simulink library "DEM_lib"  (Simulink 7.4)
settings: Solver=FixedStepDiscrete  StartTime=0.0  StopTime=Inf  FixedStep=0.001  RelTol=1e-3
undefined symbols (not defined in the file or in its folder): BCU_Drive_St, BCU_FastCharge_St, BCU_SlowCharge_St, COR_Fault_Bus, CTC_DefaultOffline_CtrCmd, CTC_DriveEmgyDcnct_CtrCmd, CTC_DriveOffline_CtrCmd, CTC_DriveOnline_CtrCmd, EHP_Fault_Bus, FCM_Fault_Bus, SCM_Fault_Bus
libraries: Defined_Functionality x82, simulink x2
(part 1 of 4)
Description:
  | $Author:Yan LiJuan$
  | $Date:2015/03/26$
  | $Revision:1.0$
settings Model: Creator=yanlijuan2  LastModifiedBy=sunsijun

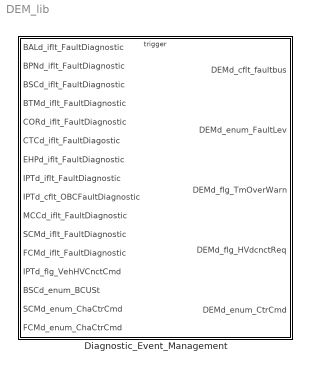
== system DEM_lib ==
  Diagnostic_Event_Management : Subsystem  TreatAsAtomicUnit=on

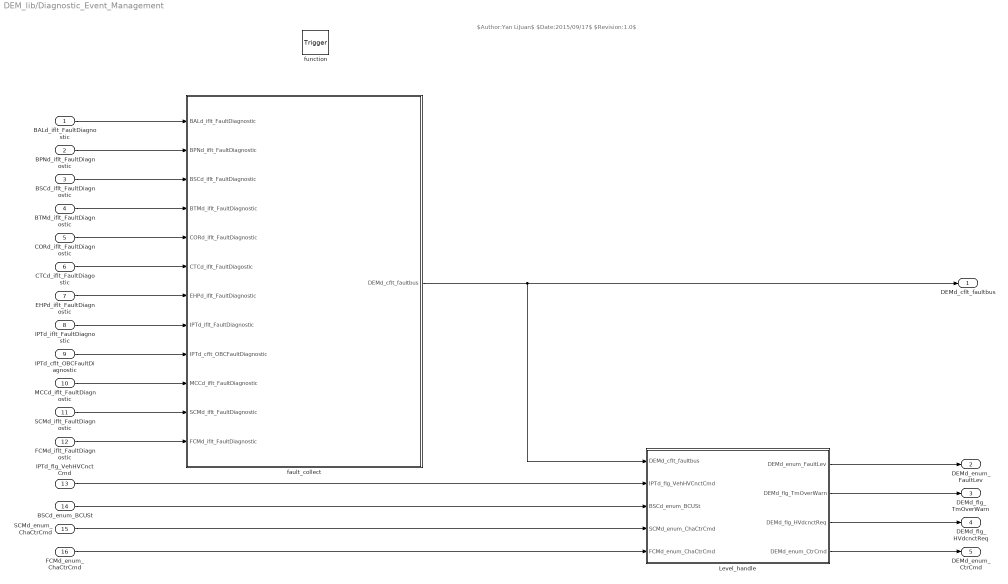
== system DEM_lib/Diagnostic_Event_Management ==
  note: $Author:Yan LiJuan$
      | $Date:2015/09/17$
      | $Revision:1.0$
  BALd_iflt_FaultDiagnostic : Inport
  BPNd_iflt_FaultDiagnostic : Inport  Port=2
  BSCd_iflt_FaultDiagnostic : Inport  Port=3
  BTMd_iflt_FaultDiagnostic : Inport  Port=4
  CORd_iflt_FaultDiagnostic : Inport  Port=5
  CTCd_iflt_FaultDiagostic : Inport  Port=6
  EHPd_iflt_FaultDiagnostic : Inport  Port=7
  IPTd_iflt_FaultDiagnostic : Inport  Port=8
  IPTd_cflt_OBCFaultDiagnostic : Inport  Port=9
  MCCd_iflt_FaultDiagnostic : Inport  Port=10
  SCMd_iflt_FaultDiagnostic : Inport  Port=11
  FCMd_iflt_FaultDiagnostic : Inport  Port=12
  IPTd_flg_VehHVCnctCmd : Inport  Port=13  DataType=boolean  OutDataTypeStr=boolean
  BSCd_enum_BCUSt : Inport  Port=14  DataType=uint8  OutDataTypeStr=uint8
  SCMd_enum_ChaCtrCmd : Inport  Port=15  DataType=uint8  OutDataTypeStr=uint8
  FCMd_enum_ChaCtrCmd : Inport  Port=16  DataType=uint8  OutDataTypeStr=uint8
  function : TriggerPort  TriggerType=function-call
  Level_handle : Subsystem  Description=|
      | $Author:Yan LiJuan$
      | $Date:2015/06/23$  
      | $Revision:1.0$
  fault_collect : Subsystem  Description=|
      | $Author:Yan LiJuan$
      | $Date:2015/06/23$  
      | $Revision:1.0$
  DEMd_cflt_faultbus : Outport  OutDataType=fixdt(1, 16)  OutScaling=2^0
  DEMd_enum_FaultLev : Outport  Port=2
  DEMd_flg_TmOverWarn : Outport  Port=3
  DEMd_flg_HVdcnctReq : Outport  Port=4
  DEMd_enum_CtrCmd : Outport  Port=5
  wires:
  IPTd_cflt_OBCFaultDiagnostic/1 -> fault_collect/9(IPTd_cflt_OBCFaultDiagnostic)
  BALd_iflt_FaultDiagnostic/1 -> fault_collect/1(BALd_iflt_FaultDiagnostic)
  BPNd_iflt_FaultDiagnostic/1 -> fault_collect/2(BPNd_iflt_FaultDiagnostic)
  BSCd_iflt_FaultDiagnostic/1 -> fault_collect/3(BSCd_iflt_FaultDiagnostic)
  BTMd_iflt_FaultDiagnostic/1 -> fault_collect/4(BTMd_iflt_FaultDiagnostic)
  CORd_iflt_FaultDiagnostic/1 -> fault_collect/5(CORd_iflt_FaultDiagnostic)
  CTCd_iflt_FaultDiagostic/1 -> fault_collect/6(CTCd_iflt_FaultDiagostic)
  fault_collect/1(DEMd_cflt_faultbus) -> DEMd_cflt_faultbus/1, Level_handle/1(DEMd_cflt_faultbus)
  EHPd_iflt_FaultDiagnostic/1 -> fault_collect/7(EHPd_iflt_FaultDiagnostic)
  IPTd_iflt_FaultDiagnostic/1 -> fault_collect/8(IPTd_iflt_FaultDiagnostic)
  MCCd_iflt_FaultDiagnostic/1 -> fault_collect/10(MCCd_iflt_FaultDiagnostic)
  SCMd_iflt_FaultDiagnostic/1 -> fault_collect/11(SCMd_iflt_FaultDiagnostic)
  FCMd_iflt_FaultDiagnostic/1 -> fault_collect/12(FCMd_iflt_FaultDiagnostic)
  Level_handle/1(DEMd_enum_FaultLev) -> DEMd_enum_FaultLev/1
  Level_handle/2(DEMd_flg_TmOverWarn) -> DEMd_flg_TmOverWarn/1
  IPTd_flg_VehHVCnctCmd/1 -> Level_handle/2(IPTd_flg_VehHVCnctCmd)
  Level_handle/3(DEMd_flg_HVdcnctReq) -> DEMd_flg_HVdcnctReq/1
  BSCd_enum_BCUSt/1 -> Level_handle/3(BSCd_enum_BCUSt)
  Level_handle/4(DEMd_enum_CtrCmd) -> DEMd_enum_CtrCmd/1
  SCMd_enum_ChaCtrCmd/1 -> Level_handle/4(SCMd_enum_ChaCtrCmd)
  FCMd_enum_ChaCtrCmd/1 -> Level_handle/5(FCMd_enum_ChaCtrCmd)

== system DEM_lib/Diagnostic_Event_Management/Level_handle ==
  DEMd_cflt_faultbus : Inport
  IPTd_flg_VehHVCnctCmd : Inport  Port=2  DataType=boolean  OutDataTypeStr=boolean
  BSCd_enum_BCUSt : Inport  Port=3  DataType=uint8  OutDataTypeStr=uint8
  SCMd_enum_ChaCtrCmd : Inport  Port=4  DataType=uint8  OutDataTypeStr=uint8
  FCMd_enum_ChaCtrCmd : Inport  Port=5  DataType=uint8  OutDataTypeStr=uint8
  CtrCmdSelect : Subsystem  Description=|
      | $Author:Yan LiJuan$
      | $Date:2015/03/26$  
      | $Revision:1.0$
  DRIVE : Subsystem  Description=|
      | $Author:Yan LiJuan$
      | $Date:2015/03/26$  
      | $Revision:1.0$
  DEMd_enum_FaultLev : Outport
  DEMd_flg_TmOverWarn : Outport  Port=2
  DEMd_flg_HVdcnctReq : Outport  Port=3
  DEMd_enum_CtrCmd : Outport  Port=4
  wires:
  DRIVE/3(DEMd_flg_HVdcnctReq) -> DEMd_flg_HVdcnctReq/1
  DRIVE/4(DEMd_enum_DrvCtrCmdRaw) -> CtrCmdSelect/1(DEMd_enum_DrvCtrCmd)
  DRIVE/2(DEMd_flg_TmOverWarn) -> DEMd_flg_TmOverWarn/1
  FCMd_enum_ChaCtrCmd/1 -> CtrCmdSelect/4(FCHMd_enum_ChaCtrCmd)
  SCMd_enum_ChaCtrCmd/1 -> CtrCmdSelect/3(SCMd_enum_ChaCtrCmd)
  CtrCmdSelect/1(DEMd_enum_CtrCmd) -> DEMd_enum_CtrCmd/1
  DRIVE/1(DEMd_enum_FaultLev) -> DEMd_enum_FaultLev/1
  BSCd_enum_BCUSt/1 -> DRIVE/3(BSCd_enum_BCUSt), CtrCmdSelect/2(BSCd_enum_BCUSt)
  IPTd_flg_VehHVCnctCmd/1 -> DRIVE/2(IPTd_flg_VehHVCnctCmd)
  DEMd_cflt_faultbus/1 -> DRIVE/1(DEMd_cflt_fault)

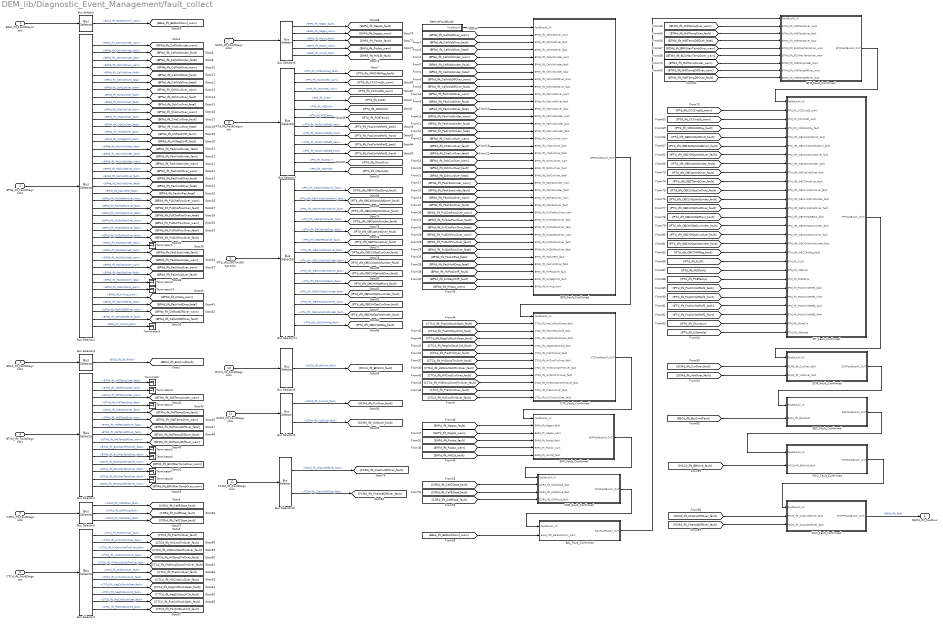
== system DEM_lib/Diagnostic_Event_Management/fault_collect ==
  BALd_iflt_FaultDiagnostic : Inport
  BPNd_iflt_FaultDiagnostic : Inport  Port=2
  BSCd_iflt_FaultDiagnostic : Inport  Port=3
  BTMd_iflt_FaultDiagnostic : Inport  Port=4
  CORd_iflt_FaultDiagnostic : Inport  Port=5
  CTCd_iflt_FaultDiagostic : Inport  Port=6
  EHPd_iflt_FaultDiagnostic : Inport  Port=7
  IPTd_iflt_FaultDiagnostic : Inport  Port=8
  IPTd_cflt_OBCFaultDiagnostic : Inport  Port=9
  MCCd_iflt_FaultDiagnostic : Inport  Port=10
  SCMd_iflt_FaultDiagnostic : Inport  Port=11
  FCMd_iflt_FaultDiagnostic : Inport  Port=12
  BAL_Fault_Confirmed : Subsystem  Description=|
      | $Author:Yan LiJuan$
      | $Date:2015/03/26$  
      | $Revision:1.0$
  BPN_Fault_Confirmed : Subsystem  Description=|
      | $Author:Yan LiJuan$
      | $Date:2015/03/26$  
      | $Revision:1.0$
  BSC_Fault_Confirmed : Subsystem  Description=|
      | $Author:Yan LiJuan$
      | $Date:2015/03/26$  
      | $Revision:1.0$
  BTM_Fault_Confirmed : Subsystem  Description=|
      | $Author:Yan LiJuan$
      | $Date:2015/03/26$  
      | $Revision:1.0$
  Bus Selector : BusSelector  OutputSignals=BALd_iflt_BalSwthAnml_warn
  Bus Selector1 : BusSelector  OutputSignals=CTCd_iflt_PrecTmOver_fault,CTCd_iflt_HVCnctTmOver_fault,CTCd_iflt_HVDcncWaitTmOver_fault,CTCd_iflt_HVDcnctTmOver_fault,CTCd_iflt_HVEmcyDcnctTmOver_fault,CTCd_iflt_PrecCurOver_fault,CTCd_iflt_HVCnctCurOver_fault,CTCd_iflt_NegCtrStuckOpen_fault,CTCd_iflt_NegCtrStuckCld_fault,CTCd_iflt_PosCtrStuckOpen_fault,CTCd_iflt_PosCtrStuckCld_fault
  Bus Selector10 : BusSelector  OutputSignals=FCMd_iflt_ChaCurDifOver_fault,FCMd_iflt_ChaVoltDifOver_fault
  Bus Selector11 : BusSelector  OutputSignals=IPTd_cflt_OBCHVOptDcnct_fault,IPTd_cflt_OBCAVOptVoltAbnml_fault,IPTd_cflt_OBCHVOptVoltOver_fault,IPTd_cflt_OBCIptVoltUnder_fault,IPTd_cflt_OBCIptVoltOver_fault,IPTd_cflt_OBCTempOver_fault,IPTd_cflt_OBCLVOptCurOver_fault,IPTd_cflt_OBCLVOptVoltUnder_fault,IPTd_cflt_OBCLVOptVoltOver_fault,IPTd_cflt_OBCHVOptRevs_fault,IPTd_cflt_OBCHVOptCurUnder_fault,IPTd_cflt_OBCHVOptCurOver_fault,IPTd_cflt_OBCHVOptVoltUnder_fault,IPTd_cflt_OBCCANMsg_fault
  Bus Selector2 : BusSelector  OutputSignals=BPNd_iflt_CellVoltDiag.BPNd_iflt_CellVoltUnder_warn,BPNd_iflt_CellVoltDiag.BPNd_iflt_CellVoltUnder_fault,BPNd_iflt_CellVoltDiag.BPNd_iflt_CellVoltUnder_fatal,BPNd_iflt_CellVoltDiag.BPNd_iflt_CellVoltOver_warn,BPNd_iflt_CellVoltDiag.BPNd_iflt_CellVoltOver_fault,BPNd_iflt_CellVoltDiag.BPNd_iflt_CellVoltOver_fatal,BPNd_iflt_ActCurDiag.BPNd_iflt_DchCurOver_warn,BPNd_iflt_ActCurDiag.BPNd_iflt_DchCurOver_fault,BPNd_iflt_ActCurDiag.BPNd_iflt_DchCurOver_fatal,BPNd_iflt_ActCurDiag.BPNd_iflt_ChaCurOver_warn,BPNd_iflt_ActCurDiag.BPNd_iflt_ChaCurOver_fault,BPNd_iflt_ActCurDiag.BPNd_iflt_ChaCurOver_fatal,BPNd_iflt_HVCtrRDiag.BPNd_iflt_HVPosCtrlR_fault,BPNd_iflt_HVCtrRDiag.BPNd_iflt_HVNegCtrlR_fault,BPNd_iflt_HighVoltDiag.BPNd_iflt_PackVoltUnder_fatal,BPNd_iflt_HighVoltDiag.BPNd_iflt_PackVoltUnder_fault,BPNd_iflt_HighVoltDiag.BPNd_iflt_PackVoltUnder_warn,BPNd_iflt_HighVoltDiag.BPNd_iflt_PackVoltOver_warn,BPNd_iflt_HighVoltDiag.BPNd_iflt_PackVoltOver_fault,BPNd_iflt_HighVoltDiag.BPNd_iflt_PackVoltOver_fatal,BPNd_iflt_PackInResDiag.BPNd_iflt_PackInRes_fatal,BPNd_iflt_ActPowDiag.BPNd_iflt_PulChaPowOver_warn,BPNd_iflt_ActPowDiag.BPNd_iflt_PulChaPowOver_fault,BPNd_iflt_ActPowDiag.BPNd_iflt_PulChaPowOver_fatal,BPNd_iflt_ActPowDiag.BPNd_iflt_PulDchPowOver_warn,BPNd_iflt_ActPowDiag.BPNd_iflt_PulDchPowOver_fatal,BPNd_iflt_ActPowDiag.BPNd_iflt_PulDchPowOver_fault,BPNd_iflt_SOCDiag.BPNd_iflt_PackSocUnder_fatal,BPNd_iflt_SOCDiag.BPNd_iflt_PackSocUnder_fault,BPNd_iflt_SOCDiag.BPNd_iflt_PackSocUnder_warn,BPNd_iflt_SOCDiag.BPNd_iflt_PackSocOver_warn,BPNd_iflt_SOCDiag.BPNd_iflt_PackSocOver_fault,BPNd_iflt_SOCDiag.BPNd_iflt_PackSocOver_fatal,BPNd_iflt_VoltAcqDiag.BPNd_iflt_MSDVoltAcq_warn,BPNd_iflt_VoltAcqDiag.BPNd_iflt_HVAcq_warn,BPNd_ilft_PackVoltDropDiag.BPNd_ilft_PackVoltDrop_fatal,BPNd_iflt_CellVoltDifDiag.BPNd_iflt_CellVoltDifOver_warn,BPNd_iflt_CellVoltDifDiag.BPNd_iflt_CellVoltDifOver_fault,BPNd_iflt_CurAcqDiag.BPNd_iflt_CurAcq_fault
  Bus Selector3 : BusSelector  OutputSignals=BSCd_iflt_BCUFault
  Bus Selector4 : BusSelector  OutputSignals=BTMd_iflt_MdlTempUnder_fatal,BTMd_iflt_MdlTempUnder_fault,BTMd_iflt_MdlTempUnder_warn,BTMd_iflt_MdlTempOver_fatal,BTMd_iflt_MdlTempOver_fault,BTMd_iflt_MdlTempOver_warn,BTMd_iflt_MdlTempDifOver_fatal,BTMd_iflt_MdlTempDifOver_fault,BTMd_iflt_MdlTempDifOver_warn,BTMd_iflt_BCUMaxTempOver_fatal,BTMd_iflt_BCUMaxTempOver_fault,BTMd_iflt_BCUMaxTempOver_warn,BTMd_iflt_BMUMaxTempOver_fatal,BTMd_iflt_BMUMaxTempOver_fault,BTMd_iflt_BMUMaxTempOver_warn
  Bus Selector5 : BusSelector  OutputSignals=CORd_iflt_CellRDcse_fault,CORd_iflt_CellRIcse_fault,CORd_iflt_CellCDcse_fault
  Bus Selector6 : BusSelector  OutputSignals=EHPd_iflt_NegIso_fault,EHPd_iflt_NegIso_warn,EHPd_iflt_PosIso_fault,EHPd_iflt_PosIso_warn,EHPd_iflt_HVILSt_fault
  Bus Selector7 : BusSelector  OutputSignals=IPTd_iflt_VMSCANMsg_fault,IPTd_iflt_CC2CnctSt_warn,IPTd_iflt_CCCnctSt_warn,IPTd_iflt_AnalogDiagnostic.IPTd_iflt_KL30,IPTd_iflt_AnalogDiagnostic.IPTd_iflt_MSDVolt,IPTd_iflt_AnalogDiagnostic.IPTd_iflt_PCBTemp,IPTd_iflt_AnalogDiagnostic.IPTd_iflt_PosCtrVoltRef1_back,IPTd_iflt_AnalogDiagnostic.IPTd_iflt_PosCtrVoltRef1_front,IPTd_iflt_AnalogDiagnostic.IPTd_iflt_PosCtrVoltRef2_back,IPTd_iflt_AnalogDiagnostic.IPTd_iflt_PosCtrVoltRef2_front,IPTd_iflt_AnalogDiagnostic.IPTd_iflt_ShuntCur,IPTd_iflt_AnalogDiagnostic.IPTd_iflt_USample
  Bus Selector8 : BusSelector  OutputSignals=MCCd_iflt_BMUInit_fault
  Bus Selector9 : BusSelector  OutputSignals=SCMd_iflt_CurOver_fault,SCMd_iflt_VoltOver_fault
  COR_Fault_Confirmed : Subsystem  Description=|
      | $Author:Yan LiJuan$
      | $Date:2015/03/26$  
      | $Revision:1.0$
  CTC_Fault_Confirmed : Subsystem  Description=|
      | $Author:Yan LiJuan$
      | $Date:2015/03/26$  
      | $Revision:1.0$
  DefaultFaultBusAll : Subsystem  Description=|
      | $Author:Yan LiJuan$
      | $Date:2015/03/26$  
      | $Revision:1.0$
  EHP_Fault_Confirmed : Subsystem  Description=|
      | $Author:Yan LiJuan$
      | $Date:2015/03/26$  
      | $Revision:1.0$
  FCM_Fault_Confirmed : Subsystem  Description=|
      | $Author:Yan LiJuan$
      | $Date:2015/03/26$  
      | $Revision:1.0$
  IPT_Fault_Confirmed : Subsystem  Description=|
      | $Author:Yan LiJuan$
      | $Date:2015/03/26$  
      | $Revision:1.0$
  MCC_Fault_Confirmed : Subsystem  Description=|
      | $Author:Yan LiJuan$
      | $Date:2015/03/26$  
      | $Revision:1.0$
  SCM_Fault_Confirmed : Subsystem  Description=|
      | $Author:Yan LiJuan$
      | $Date:2015/03/26$  
      | $Revision:1.0$
  Terminator{,1..10} (11 alike) : Terminator
  DEMd_cflt_faultbus : Outport  OutDataType=fixdt(1, 16)  OutScaling=2^0
  wires:
  Bus Selector2/39 -> Terminator9/1  "<BPNd_iflt_CurAcq_fault>"
  Bus Selector2/35 -> [BPNd_iflt_HVAcq_warn]  "<BPNd_iflt_HVAcq_warn>"
  [IPTd_cflt_OBCHVOptDcnct_fault] -> IPT_Fault_Confirmed/5(IPTd_cflt_OBCHVOptDcnct_fault)
  [IPTd_cflt_OBCAVOptVoltAbnml_fault] -> IPT_Fault_Confirmed/6(IPTd_cflt_OBCAVOptVoltAbnml_fault)
  Bus Selector11/14 -> [IPTd_cflt_OBCCANMsg_fault]  "<IPTd_cflt_OBCCANMsg_fault>"
  Bus Selector11/13 -> [IPTd_cflt_OBCHVOptVoltUnder_fault]  "<IPTd_cflt_OBCHVOptVoltUnder_fault>"
  Bus Selector11/12 -> [IPTd_cflt_OBCHVOptCurOver_fault]  "<IPTd_cflt_OBCHVOptCurOver_fault>"
  Bus Selector11/11 -> [IPTd_cflt_OBCHVOptCurUnder_fault]  "<IPTd_cflt_OBCHVOptCurUnder_fault>"
  Bus Selector11/10 -> [IPTd_cflt_OBCHVOptRevs_fault]  "<IPTd_cflt_OBCHVOptRevs_fault>"
  Bus Selector11/9 -> [IPTd_cflt_OBCLVOptVoltOver_fault]  "<IPTd_cflt_OBCLVOptVoltOver_fault>"
  Bus Selector11/8 -> [IPTd_cflt_OBCLVOptVoltUnder_fault]  "<IPTd_cflt_OBCLVOptVoltUnder_fault>"
  Bus Selector11/7 -> [IPTd_cflt_OBCLVOptCurOver_fault]  "<IPTd_cflt_OBCLVOptCurOver_fault>"
  Bus Selector11/6 -> [IPTd_cflt_OBCTempOver_fault]  "<IPTd_cflt_OBCTempOver_fault>"
  Bus Selector11/5 -> [IPTd_cflt_OBCIptVoltOver_fault]  "<IPTd_cflt_OBCIptVoltOver_fault>"
  Bus Selector11/4 -> [IPTd_cflt_OBCIptVoltUnder_fault]  "<IPTd_cflt_OBCIptVoltUnder_fault>"
  Bus Selector11/3 -> [IPTd_cflt_OBCHVOptVoltOver_fault]  "<IPTd_cflt_OBCHVOptVoltOver_fault>"
  Bus Selector11/2 -> [IPTd_cflt_OBCAVOptVoltAbnml_fault]  "<IPTd_cflt_OBCAVOptVoltAbnml_fault>"
  Bus Selector11/1 -> [IPTd_cflt_OBCHVOptDcnct_fault]  "<IPTd_cflt_OBCHVOptDcnct_fault>"
  Bus Selector7/12 -> [IPTd_iflt_USample]  "<IPTd_iflt_USample>"
  Bus Selector7/11 -> [IPTd_iflt_ShuntCur]  "<IPTd_iflt_ShuntCur>"
  Bus Selector7/10 -> [IPTd_iflt_PosCtrVoltRef2_front]  "<IPTd_iflt_PosCtrVoltRef2_front>"
  Bus Selector7/9 -> [IPTd_iflt_PosCtrVoltRef2_back]  "<IPTd_iflt_PosCtrVoltRef2_back>"
  Bus Selector7/8 -> [IPTd_iflt_PosCtrVoltRef1_front]  "<IPTd_iflt_PosCtrVoltRef1_front>"
  Bus Selector7/7 -> [IPTd_iflt_PosCtrVoltRef1_back]  "<IPTd_iflt_PosCtrVoltRef1_back>"
  Bus Selector7/6 -> [IPTd_iflt_PCBTemp]  "<IPTd_iflt_PCBTemp>"
  Bus Selector7/5 -> [IPTd_iflt_MSDVolt]  "<IPTd_iflt_MSDVolt>"
  Bus Selector7/4 -> [IPTd_iflt_KL30]  "<IPTd_iflt_KL30>"
  Bus Selector7/3 -> [IPTd_iflt_CCCnctSt_warn]  "<IPTd_iflt_CCCnctSt_warn>"
  Bus Selector7/2 -> [IPTd_iflt_CC2CnctSt_warn]  "<IPTd_iflt_CC2CnctSt_warn>"
  Bus Selector7/1 -> [IPTd_iflt_VMSCANMsg_fault]  "<IPTd_iflt_VMSCANMsg_fault>"
  IPTd_cflt_OBCFaultDiagnostic/1 -> Bus Selector11/1
  FCM_Fault_Confirmed/1(FCMIPTFaultBusAll_OUT) -> DEMd_cflt_faultbus/1  "DEMd_cflt_fault"
  [FCMd_iflt_ChaVoltDifOver_fault] -> FCM_Fault_Confirmed/3(FCMd_iflt_ChaVoltDifOver_fault)
  [FCMd_iflt_ChaCurDifOver_fault] -> FCM_Fault_Confirmed/2(FCMd_iflt_ChaCurDifOver_fault)
  Bus Selector10/2 -> [FCMd_iflt_ChaVoltDifOver_fault]  "<FCMd_iflt_ChaVoltDifOver_fault>"
  Bus Selector10/1 -> [FCMd_iflt_ChaCurDifOver_fault]  "<FCMd_iflt_ChaCurDifOver_fault>"
  FCMd_iflt_FaultDiagnostic/1 -> Bus Selector10/1
  [BSCd_iflt_BcuCmdFault] -> BSC_Fault_Confirmed/2(BSCd_iflt_BCUFault)
  BSC_Fault_Confirmed/1(BSCFaultBusAll_OUT) -> MCC_Fault_Confirmed/1(FaultBusAll_IN)
  SCM_Fault_Confirmed/1(SCMFaultBusAll_OUT) -> BSC_Fault_Confirmed/1(FaultBusAll_IN)
  [SCMd_iflt_VoltOver_fault] -> SCM_Fault_Confirmed/3(SCMd_iflt_VoltOver_fault)
  [SCMd_iflt_CurOver_fault] -> SCM_Fault_Confirmed/2(SCMd_iflt_CurOver_fault)
  Bus Selector9/2 -> [SCMd_iflt_VoltOver_fault]  "<SCMd_iflt_VoltOver_fault>"
  SCMd_iflt_FaultDiagnostic/1 -> Bus Selector9/1
  Bus Selector9/1 -> [SCMd_iflt_CurOver_fault]  "<SCMd_iflt_CurOver_fault>"
  [IPTd_cflt_OBCCANMsg_fault] -> IPT_Fault_Confirmed/18(IPTd_cflt_OBCCANMsg_fault)
  [IPTd_cflt_OBCHVOptVoltUnder_fault] -> IPT_Fault_Confirmed/17(IPTd_cflt_OBCHVOptVoltUnder_fault)
  [IPTd_cflt_OBCHVOptCurOver_fault] -> IPT_Fault_Confirmed/16(IPTd_cflt_OBCHVOptCurOver_fault)
  [IPTd_cflt_OBCHVOptCurUnder_fault] -> IPT_Fault_Confirmed/15(IPTd_cflt_OBCHVOptCurUnder_fault)
  [IPTd_cflt_OBCHVOptRevs_fault] -> IPT_Fault_Confirmed/14(IPTd_cflt_OBCHVOptRevs_fault)
  [IPTd_cflt_OBCLVOptVoltOver_fault] -> IPT_Fault_Confirmed/13(IPTd_cflt_OBCLVOptVoltOver_fault)
  [IPTd_cflt_OBCLVOptVoltUnder_fault] -> IPT_Fault_Confirmed/12(IPTd_cflt_OBCLVOptVoltUnder_fault)
  [IPTd_cflt_OBCLVOptCurOver_fault] -> IPT_Fault_Confirmed/11(IPTd_cflt_OBCLVOptCurOver_fault)
  [IPTd_cflt_OBCTempOver_fault] -> IPT_Fault_Confirmed/10(IPTd_cflt_OBCTempOver_fault)
  [IPTd_cflt_OBCIptVoltOver_fault] -> IPT_Fault_Confirmed/9(IPTd_cflt_OBCIptVoltOver_fault)
  [IPTd_cflt_OBCIptVoltUnder_fault] -> IPT_Fault_Confirmed/8(IPTd_cflt_OBCIptVoltUnder_fault)
  [IPTd_cflt_OBCHVOptVoltOver_fault] -> IPT_Fault_Confirmed/7(IPTd_cflt_OBCHVOptVoltOver_fault)
  [CTCd_iflt_HVCnctCurOver_fault] -> CTC_Fault_Confirmed/9(CTCd_iflt_HVDcnctTmOver_fault)
  [CTCd_iflt_HVCnctTmOver_fault] -> CTC_Fault_Confirmed/12(CTCd_iflt_HVCnctCurOver_fault)
  [CTCd_iflt_PrecCurOver_fault] -> CTC_Fault_Confirmed/11(CTCd_iflt_PrecCurOver_fault)
  [CTCd_iflt_HVEmcyDcnctTmOver_fault] -> CTC_Fault_Confirmed/10(CTCd_iflt_HVEmcyDcnctTmOver_fault)
  [CTCd_iflt_HVDcncWaitTmOver_fault] -> CTC_Fault_Confirmed/8(CTCd_iflt_HVDcncWaitTmOver_fault)
  [CTCd_iflt_HVDcnctTmOver_fault] -> CTC_Fault_Confirmed/7(CTCd_iflt_HVCnctTmOver_fault)
  [CTCd_iflt_PrecTmOver_fault] -> CTC_Fault_Confirmed/6(CTCd_iflt_PrecTmOver_fault)
  [CTCd_iflt_NegCtrStuckCld_fault] -> CTC_Fault_Confirmed/5(CTCd_iflt_NegCtrStuckCld_fault)
  [CTCd_iflt_NegCtrStuckOpen_fault] -> CTC_Fault_Confirmed/4(CTCd_iflt_NegCtrStuckOpen_fault)
  [CTCd_iflt_PosCtrStuckCld_fault] -> CTC_Fault_Confirmed/3(CTCd_iflt_PosCtrStuckCld_fault)
  [CTCd_iflt_PosCtrStuckOpen_fault] -> CTC_Fault_Confirmed/2(CTCd_iflt_PosCtrStuckOpen_fault)
  [BTMd_iflt_MdlTempUnder_warn] -> BTM_Fault_Confirmed/7(BTMd_iflt_MdlTempUnder_warn)
  [BTMd_iflt_BMUMaxTempOver_warn] -> BTM_Fault_Confirmed/5(BTMd_iflt_BMUMaxTempOver_warn)
  [BTMd_iflt_BCUMaxTempOver_warn] -> BTM_Fault_Confirmed/6(BTMd_iflt_BCUMaxTempOver_warn)
  [BTMd_iflt_MdlTempDifOver_fatal] -> BTM_Fault_Confirmed/4(BTMd_iflt_MdlTempOver_fatal)
  [BTMd_iflt_MdlTempOver_fault] -> BTM_Fault_Confirmed/3(BTMd_iflt_MdlTempOver_fault)
  [BTMd_iflt_MdlTempOver_warn] -> BTM_Fault_Confirmed/2(BTMd_iflt_MdlTempOver_warn)
  [EHPd_iflt_HVILSt_fault] -> EHP_Fault_Confirmed/6(EHPd_iflt_HVILSt_fault)
  IPT_Fault_Confirmed/1(IPTFaultBusAll_OUT) -> SCM_Fault_Confirmed/1(FaultBusAll_IN)
  BTM_Fault_Confirmed/1(BTMFaultBusAll_OUT) -> IPT_Fault_Confirmed/1(FaultBusAll_IN)
  BAL_Fault_Confirmed/1(BALFaultBusAll_OUT) -> BTM_Fault_Confirmed/1(FaultBusAll_IN)
  COR_Fault_Confirmed/1(CORFaultBusAll_OUT) -> BAL_Fault_Confirmed/1(FaultBusAll_IN)
  EHP_Fault_Confirmed/1(EHPFaultBusAll_OUT) -> COR_Fault_Confirmed/1(FaultBusAll_IN)
  [BALd_iflt_BalSwthAnml_warn] -> BAL_Fault_Confirmed/2(BALd_iflit_BalSwthAnml_warn)
  BPN_Fault_Confirmed/1(BPNFaultBusAll_OUT) -> CTC_Fault_Confirmed/1(FaultBusAll_IN)
  CTC_Fault_Confirmed/1(CTCFaultBusAll_OUT) -> EHP_Fault_Confirmed/1(FaultBusAll_IN)
  DefaultFaultBusAll/1(FaultBusAll) -> BPN_Fault_Confirmed/1(FaultBusAll_IN)
  BSCd_iflt_FaultDiagnostic/1 -> Bus Selector3/1
  BTMd_iflt_FaultDiagnostic/1 -> Bus Selector4/1
  CORd_iflt_FaultDiagnostic/1 -> Bus Selector5/1
  CTCd_iflt_FaultDiagostic/1 -> Bus Selector1/1
  MCCd_iflt_FaultDiagnostic/1 -> Bus Selector8/1
  BPNd_iflt_FaultDiagnostic/1 -> Bus Selector2/1
  BALd_iflt_FaultDiagnostic/1 -> Bus Selector/1
  Bus Selector/1 -> [BALd_iflt_BalSwthAnml_warn]  "<BALd_iflt_BalSwthAnml_warn>"
  Bus Selector2/1 -> [BPNd_iflt_CellVoltUnder_warn]  "<BPNd_iflt_CellVoltUnder_warn>"
  Bus Selector2/2 -> [BPNd_iflt_CellVoltUnder_fault]  "<BPNd_iflt_CellVoltUnder_fault>"
  Bus Selector2/3 -> [BPNd_iflt_CellVoltUnder_fatal]  "<BPNd_iflt_CellVoltUnder_fatal>"
  Bus Selector2/4 -> [BPNd_iflt_CellVoltOver_warn]  "<BPNd_iflt_CellVoltOver_warn>"
  Bus Selector2/5 -> [BPNd_iflt_CellVoltOver_fault]  "<BPNd_iflt_CellVoltOver_fault>"
  Bus Selector2/6 -> [BPNd_iflt_CellVoltOver_fatal]  "<BPNd_iflt_CellVoltOver_fatal>"
  Bus Selector2/7 -> [BPNd_iflt_DchCurOver_warn]  "<BPNd_iflt_DchCurOver_warn>"
  Bus Selector2/8 -> [BPNd_iflt_DchCurOver_fault]  "<BPNd_iflt_DchCurOver_fault>"
  Bus Selector2/9 -> [BPNd_iflt_DchCurOver_fatal]  "<BPNd_iflt_DchCurOver_fatal>"
  Bus Selector2/10 -> [BPNd_iflt_ChaCurOver_warn]  "<BPNd_iflt_ChaCurOver_warn>"
  Bus Selector2/11 -> [BPNd_iflt_ChaCurOver_fault]  "<BPNd_iflt_ChaCurOver_fault>"
  Bus Selector2/12 -> [BPNd_iflt_ChaCurOver_fatal]  "<BPNd_iflt_ChaCurOver_fatal>"
  Bus Selector2/13 -> [BPNd_iflt_HVPosCtrlR_fault]  "<BPNd_iflt_HVPosCtrlR_fault>"
  Bus Selector2/14 -> [BPNd_iflt_HVNegCtrlR_fault]  "<BPNd_iflt_HVNegCtrlR_fault>"
  Bus Selector2/15 -> [BPNd_iflt_PackVoltUnder_fatal]  "<BPNd_iflt_PackVoltUnder_fatal>"
  Bus Selector2/16 -> [BPNd_iflt_PackVoltUnder_fault]  "<BPNd_iflt_PackVoltUnder_fault>"
  Bus Selector2/17 -> [BPNd_iflt_PackVoltUnder_warn]  "<BPNd_iflt_PackVoltUnder_warn>"
  Bus Selector2/18 -> [BPNd_iflt_PackVoltOver_warn]  "<BPNd_iflt_PackVoltOver_warn>"
  Bus Selector2/19 -> [BPNd_iflt_PackVoltOver_fault]  "<BPNd_iflt_PackVoltOver_fault>"
  Bus Selector2/20 -> [BPNd_iflt_PackVoltOver_fatal]  "<BPNd_iflt_PackVoltOver_fatal>"
  Bus Selector2/21 -> [BPNd_iflt_PackInRes_fatal]  "<BPNd_iflt_PackInRes_fatal>"
  Bus Selector2/22 -> [BPNd_iflt_PulChaPowOver_warn]  "<BPNd_iflt_PulChaPowOver_warn>"
  Bus Selector2/23 -> [BPNd_iflt_PulChaPowOver_fault]  "<BPNd_iflt_PulChaPowOver_fault>"
  Bus Selector2/24 -> [BPNd_iflt_PulChaPowOver_fatal]  "<BPNd_iflt_PulChaPowOver_fatal>"
  Bus Selector2/25 -> [BPNd_iflt_PulDchPowOver_warn]  "<BPNd_iflt_PulDchPowOver_warn>"
  Bus Selector2/27 -> [BPNd_iflt_PulDchPowOver_fault]  "<BPNd_iflt_PulDchPowOver_fault>"
  Bus Selector2/26 -> [BPNd_iflt_PulDchPowOver_fatal]  "<BPNd_iflt_PulDchPowOver_fatal>"
  Bus Selector2/30 -> [BPNd_iflt_PackSocUnder_warn]  "<BPNd_iflt_PackSocUnder_warn>"
  Bus Selector2/29 -> [BPNd_iflt_PackSocUnder_fault]  "<BPNd_iflt_PackSocUnder_fault>"
  Bus Selector2/28 -> Terminator1/1  "<BPNd_iflt_PackSocUnder_fatal>"
  Bus Selector2/31 -> [BPNd_iflt_PackSocOver_warn]  "<BPNd_iflt_PackSocOver_warn>"
  Bus Selector2/32 -> [BPNd_iflt_PackSocOver_fault]  "<BPNd_iflt_PackSocOver_fault>"
  Bus Selector2/33 -> Terminator2/1  "<BPNd_iflt_PackSocOver_fatal>"
  Bus Selector2/34 -> Terminator10/1  "<BPNd_iflt_MSDVoltAcq_warn>"
  Bus Selector2/36 -> [BPNd_ilft_PackVoltDrop_fatal]  "<BPNd_ilft_PackVoltDrop_fatal>"
  Bus Selector3/1 -> [BSCd_iflt_BcuCmdFault]  "<BSCd_iflt_BCUFault>"
  Bus Selector4/1 -> Terminator/1  "<BTMd_iflt_MdlTempUnder_fatal>"
  Bus Selector4/2 -> Terminator3/1  "<BTMd_iflt_MdlTempUnder_fault>"
  Bus Selector4/3 -> [BTMd_iflt_MdlTempUnder_warn]  "<BTMd_iflt_MdlTempUnder_warn>"
  Bus Selector4/4 -> Terminator4/1  "<BTMd_iflt_MdlTempOver_fatal>"
  Bus Selector4/5 -> [BTMd_iflt_MdlTempOver_fault]  "<BTMd_iflt_MdlTempOver_fault>"
  Bus Selector4/6 -> [BTMd_iflt_MdlTempOver_warn]  "<BTMd_iflt_MdlTempOver_warn>"
  Bus Selector4/7 -> [BTMd_iflt_MdlTempDifOver_fatal]  "<BTMd_iflt_MdlTempDifOver_fatal>"
  Bus Selector4/8 -> [BTMd_iflt_MdlTempDifOver_fault]  "<BTMd_iflt_MdlTempDifOver_fault>"
  Bus Selector4/9 -> [BTMd_iflt_MdlTempDifOver_warn]  "<BTMd_iflt_MdlTempDifOver_warn>"
  Bus Selector4/10 -> Terminator5/1  "<BTMd_iflt_BCUMaxTempOver_fatal>"
  Bus Selector4/11 -> Terminator6/1  "<BTMd_iflt_BCUMaxTempOver_fault>"
  Bus Selector4/12 -> [BTMd_iflt_BCUMaxTempOver_warn]  "<BTMd_iflt_BCUMaxTempOver_warn>"
  Bus Selector4/13 -> Terminator7/1  "<BTMd_iflt_BMUMaxTempOver_fatal>"
  Bus Selector4/14 -> Terminator8/1  "<BTMd_iflt_BMUMaxTempOver_fault>"
  Bus Selector4/15 -> [BTMd_iflt_BMUMaxTempOver_warn]  "<BTMd_iflt_BMUMaxTempOver_warn>"
  Bus Selector5/1 -> [CORd_iflt_CellRDcse_fault]  "<CORd_iflt_CellRDcse_fault>"
  Bus Selector5/3 -> [CORd_iflt_CellCDcse_fault]  "<CORd_iflt_CellCDcse_fault>"
  Bus Selector5/2 -> [CORd_iflt_CellRIcse_fault]  "<CORd_iflt_CellRIcse_fault>"
  Bus Selector1/1 -> [CTCd_iflt_PrecTmOver_fault]  "<CTCd_iflt_PrecTmOver_fault>"
  Bus Selector1/2 -> [CTCd_iflt_HVCnctTmOver_fault]  "<CTCd_iflt_HVCnctTmOver_fault>"
  Bus Selector1/3 -> [CTCd_iflt_HVDcncWaitTmOver_fault]  "<CTCd_iflt_HVDcncWaitTmOver_fault>"
  Bus Selector1/4 -> [CTCd_iflt_HVDcnctTmOver_fault]  "<CTCd_iflt_HVDcnctTmOver_fault>"
  Bus Selector1/5 -> [CTCd_iflt_HVEmcyDcnctTmOver_fault]  "<CTCd_iflt_HVEmcyDcnctTmOver_fault>"
  Bus Selector1/6 -> [CTCd_iflt_PrecCurOver_fault]  "<CTCd_iflt_PrecCurOver_fault>"
  Bus Selector1/7 -> [CTCd_iflt_HVCnctCurOver_fault]  "<CTCd_iflt_HVCnctCurOver_fault>"
  Bus Selector1/8 -> [CTCd_iflt_NegCtrStuckOpen_fault]  "<CTCd_iflt_NegCtrStuckOpen_fault>"
  Bus Selector1/9 -> [CTCd_iflt_NegCtrStuckCld_fault]  "<CTCd_iflt_NegCtrStuckCld_fault>"
  Bus Selector1/10 -> [CTCd_iflt_PosCtrStuckOpen_fault]  "<CTCd_iflt_PosCtrStuckOpen_fault>"
  Bus Selector1/11 -> [CTCd_iflt_PosCtrStuckCld_fault]  "<CTCd_iflt_PosCtrStuckCld_fault>"
  EHPd_iflt_FaultDiagnostic/1 -> Bus Selector6/1
  Bus Selector6/1 -> [EHPd_iflt_NegIso_fault]  "<EHPd_iflt_NegIso_fault>"
  Bus Selector6/2 -> [EHPd_iflt_NegIso_warn]  "<EHPd_iflt_NegIso_warn>"
  Bus Selector6/3 -> [EHPd_iflt_PosIso_fault]  "<EHPd_iflt_PosIso_fault>"
  Bus Selector6/4 -> [EHPd_iflt_PosIso_warn]  "<EHPd_iflt_PosIso_warn>"
  Bus Selector6/5 -> [EHPd_iflt_HVILSt_fault]  "<EHPd_iflt_HVILSt_fault>"
  IPTd_iflt_FaultDiagnostic/1 -> Bus Selector7/1
  Bus Selector8/1 -> [MCCd_iflt_BMUInit_fault]  "<MCCd_iflt_BMUInit_fault>"
  [BPNd_iflt_CellVoltOver_warn] -> BPN_Fault_Confirmed/2(BPNd_iflt_CellVoltOver_warn)
  [BPNd_iflt_CellVoltOver_fault] -> BPN_Fault_Confirmed/3(BPNd_iflt_CellVoltOver_fault)
  [BPNd_iflt_CellVoltOver_fatal] -> BPN_Fault_Confirmed/4(BPNd_iflt_CellVoltOver_fatal)
  [BPNd_iflt_CellVoltUnder_warn] -> BPN_Fault_Confirmed/5(BPNd_iflt_CellVoltUnder_warn)
  [BPNd_iflt_CellVoltUnder_fault] -> BPN_Fault_Confirmed/6(BPNd_iflt_CellVoltUnder_fault)
  [BPNd_iflt_CellVoltUnder_fatal] -> BPN_Fault_Confirmed/7(BPNd_iflt_CellVoltUnder_fatal)
  [BPNd_iflt_CellVoltDifOver_warn] -> BPN_Fault_Confirmed/8(BPNd_iflt_CellVoltDifOver_warn)
  [BPNd_iflt_CellVoltDifOver_fault] -> BPN_Fault_Confirmed/9(BPNd_iflt_CellVoltDifOver_fault)
  [BPNd_iflt_PackVoltOver_warn] -> BPN_Fault_Confirmed/10(BPNd_iflt_PackVoltOver_warn)
  [BPNd_iflt_PackVoltOver_fault] -> BPN_Fault_Confirmed/11(BPNd_iflt_PackVoltOver_fault)
  [BPNd_iflt_PackVoltOver_fatal] -> BPN_Fault_Confirmed/12(BPNd_iflt_PackVoltOver_fatal)
  [BPNd_iflt_PackVoltUnder_warn] -> BPN_Fault_Confirmed/13(BPNd_iflt_PackVoltUnder_warn)
  [BPNd_iflt_PackVoltUnder_fault] -> BPN_Fault_Confirmed/14(BPNd_iflt_PackVoltUnder_fault)
  [BPNd_iflt_PackVoltUnder_fatal] -> BPN_Fault_Confirmed/15(BPNd_iflt_PackVoltUnder_fatal)
  [BPNd_iflt_ChaCurOver_warn] -> BPN_Fault_Confirmed/16(BPNd_iflt_ChaCurOver_warn)
  [BPNd_iflt_ChaCurOver_fault] -> BPN_Fault_Confirmed/17(BPNd_iflt_ChaCurOver_fault)
  [BPNd_iflt_ChaCurOver_fatal] -> BPN_Fault_Confirmed/18(BPNd_iflt_ChaCurOver_fatal)
  [BPNd_iflt_DchCurOver_warn] -> BPN_Fault_Confirmed/19(BPNd_iflt_DchCurOver_warn)
  [BPNd_iflt_DchCurOver_fault] -> BPN_Fault_Confirmed/20(BPNd_iflt_DchCurOver_fault)
  [BPNd_iflt_DchCurOver_fatal] -> BPN_Fault_Confirmed/21(BPNd_iflt_DchCurOver_fatal)
  [BPNd_iflt_PackSocUnder_warn] -> BPN_Fault_Confirmed/22(BPNd_iflt_PackSocUnder_warn)
  [BPNd_iflt_PackSocUnder_fault] -> BPN_Fault_Confirmed/23(BPNd_iflt_PackSocUnder_fault)
  [BPNd_iflt_PackSocOver_warn] -> BPN_Fault_Confirmed/24(BPNd_iflt_PackSocOver_warn)
  [BPNd_iflt_PackSocOver_fault] -> BPN_Fault_Confirmed/25(BPNd_iflt_PackSocOver_fault)
  [BPNd_iflt_PulChaPowOver_warn] -> BPN_Fault_Confirmed/26(BPNd_iflt_PulChaPowOver_warn)
  [BPNd_iflt_PulChaPowOver_fault] -> BPN_Fault_Confirmed/27(BPNd_iflt_PulChaPowOver_fault)
  [BPNd_iflt_PulChaPowOver_fatal] -> BPN_Fault_Confirmed/28(BPNd_iflt_PulChaPowOver_fatal)
  [BPNd_iflt_PulDchPowOver_warn] -> BPN_Fault_Confirmed/29(BPNd_iflt_PulDchPowOver_warn)
  [BPNd_iflt_PulDchPowOver_fault] -> BPN_Fault_Confirmed/30(BPNd_iflt_PulDchPowOver_fault)
  [BPNd_iflt_PulDchPowOver_fatal] -> BPN_Fault_Confirmed/31(BPNd_iflt_PulDchPowOver_fatal)
  [BPNd_iflt_PackInRes_fatal] -> BPN_Fault_Confirmed/32(BPNd_iflt_PackInRes_fatal)
  [BPNd_ilft_PackVoltDrop_fatal] -> BPN_Fault_Confirmed/33(BPNd_iflt_PackVoltDrop_fatal)
  [BPNd_iflt_HVPosCtrlR_fault] -> BPN_Fault_Confirmed/34(BPNd_iflt_HVPosCtrlR_fault)
  [BPNd_iflt_HVNegCtrlR_fault] -> BPN_Fault_Confirmed/35(BPNd_iflt_HVNegCtrlR_fault)
  [BPNd_iflt_HVAcq_warn] -> BPN_Fault_Confirmed/36(BPNd_iflt_HVAcq_warn)
  [EHPd_iflt_NegIso_fault] -> EHP_Fault_Confirmed/2(EHPd_iflt_NegIso_fault)
  [EHPd_iflt_NegIso_warn] -> EHP_Fault_Confirmed/3(EHPd_iflt_NegIso_warn)
  [EHPd_iflt_PosIso_fault] -> EHP_Fault_Confirmed/4(EHPd_iflt_PosIso_fault)
  [EHPd_iflt_PosIso_warn] -> EHP_Fault_Confirmed/5(EHPd_iflt_PosIso_warn)
  [CORd_iflt_CellCDcse_fault] -> COR_Fault_Confirmed/2(CORd_iflt_CellCDcse_fault)
  [CORd_iflt_CellRDcse_fault] -> COR_Fault_Confirmed/3(CORd_iflt_CellRDcse_fault)
  [CORd_iflt_CellRIcse_fault] -> COR_Fault_Confirmed/4(CORd_iflt_CellRIcse_fault)
  [BTMd_iflt_MdlTempDifOver_warn] -> BTM_Fault_Confirmed/8(BTMd_iflt_MdlTempDifOver_warn)
  [BTMd_iflt_MdlTempDifOver_fault] -> BTM_Fault_Confirmed/9(BTMd_iflt_MdlTempDifOver_fault)
  [IPTd_iflt_CC2CnctSt_warn] -> IPT_Fault_Confirmed/2(IPTd_iflt_CC2CnctSt_warn)
  [IPTd_iflt_CCCnctSt_warn] -> IPT_Fault_Confirmed/3(IPTd_iflt_CCCnctSt_warn)
  [IPTd_iflt_VMSCANMsg_fault] -> IPT_Fault_Confirmed/4(IPTd_iflt_VMSCANMsg_fault)
  Bus Selector2/37 -> [BPNd_iflt_CellVoltDifOver_warn]  "<BPNd_iflt_CellVoltDifOver_warn>"
  Bus Selector2/38 -> [BPNd_iflt_CellVoltDifOver_fault]  "<BPNd_iflt_CellVoltDifOver_fault>"
  [MCCd_iflt_BMUInit_fault] -> MCC_Fault_Confirmed/2(MCCd_iflt_BMUInit_fault)
  MCC_Fault_Confirmed/1(MCCFaultBusAll_OUT) -> FCM_Fault_Confirmed/1(FaultBusAll_IN)
  [IPTd_iflt_KL30] -> IPT_Fault_Confirmed/19(IPTd_iflt_KL30)
  [IPTd_iflt_MSDVolt] -> IPT_Fault_Confirmed/20(IPTd_iflt_MSDVolt)
  [IPTd_iflt_PCBTemp] -> IPT_Fault_Confirmed/21(IPTd_iflt_PCBTemp)
  [IPTd_iflt_PosCtrVoltRef1_back] -> IPT_Fault_Confirmed/22(IPTd_iflt_PosCtrVoltRef1_back)
  [IPTd_iflt_PosCtrVoltRef1_front] -> IPT_Fault_Confirmed/23(IPTd_iflt_PosCtrVoltRef1_front)
  [IPTd_iflt_PosCtrVoltRef2_back] -> IPT_Fault_Confirmed/24(IPTd_iflt_PosCtrVoltRef2_back)
  [IPTd_iflt_PosCtrVoltRef2_front] -> IPT_Fault_Confirmed/25(IPTd_iflt_PosCtrVoltRef2_front)
  [IPTd_iflt_ShuntCur] -> IPT_Fault_Confirmed/26(IPTd_iflt_ShuntCur)
  [IPTd_iflt_USample] -> IPT_Fault_Confirmed/27(IPTd_iflt_USample)

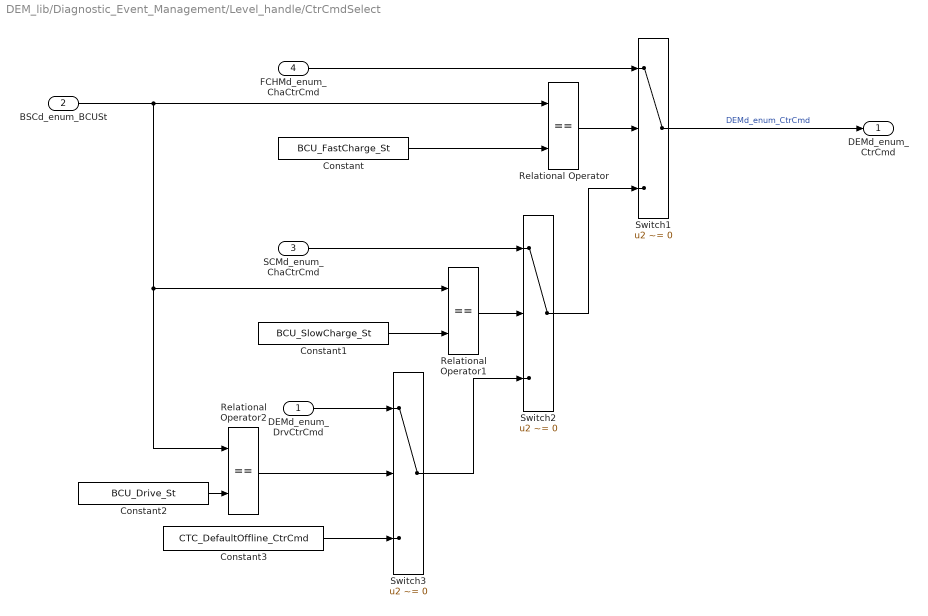
== system DEM_lib/Diagnostic_Event_Management/Level_handle/CtrCmdSelect ==
  DEMd_enum_DrvCtrCmd : Inport
  BSCd_enum_BCUSt : Inport  Port=2
  SCMd_enum_ChaCtrCmd : Inport  Port=3  OutDataType=fixdt(1, 16)  OutScaling=2^0
  FCHMd_enum_ChaCtrCmd : Inport  Port=4  OutDataType=fixdt(1, 16)  OutScaling=2^0
  Constant : Constant  Value=BCU_FastCharge_St  OutDataTypeMode=uint8  OutDataType=fixdt(1, 16)  OutScaling=2^0  OutDataTypeStr=uint8
  Constant1 : Constant  Value=BCU_SlowCharge_St  OutDataTypeMode=uint8  OutDataType=fixdt(1, 16)  OutScaling=2^0  OutDataTypeStr=uint8
  Constant2 : Constant  Value=BCU_Drive_St  OutDataTypeMode=uint8  OutDataType=fixdt(1, 16)  OutScaling=2^0  OutDataTypeStr=uint8
  Constant3 : Constant  Value=CTC_DefaultOffline_CtrCmd  OutDataTypeMode=uint8  OutDataTypeStr=uint8
  Relational Operator : RelationalOperator  Operator===  LogicOutDataTypeMode=boolean  LogicDataType=fixdt(0, 8)  OutDataTypeStr=boolean
  Relational Operator1 : RelationalOperator  Operator===  LogicOutDataTypeMode=boolean  LogicDataType=fixdt(0, 8)  OutDataTypeStr=boolean
  Relational Operator2 : RelationalOperator  Operator===  LogicOutDataTypeMode=boolean  LogicDataType=fixdt(0, 8)  OutDataTypeStr=boolean
  Switch1 : Switch  Criteria=u2 ~= 0  OutDataTypeMode=uint8  OutDataTypeStr=uint8
  Switch2 : Switch  Criteria=u2 ~= 0  OutDataTypeMode=uint8  OutDataTypeStr=uint8
  Switch3 : Switch  Criteria=u2 ~= 0  OutDataTypeMode=uint8  OutDataTypeStr=uint8
  DEMd_enum_CtrCmd : Outport
  wires:
  Constant2/1 -> Relational Operator2/2
  Relational Operator2/1 -> Switch3/2
  SCMd_enum_ChaCtrCmd/1 -> Switch2/1
  FCHMd_enum_ChaCtrCmd/1 -> Switch1/1
  Constant3/1 -> Switch3/3
  Constant1/1 -> Relational Operator1/2
  Relational Operator1/1 -> Switch2/2
  Constant/1 -> Relational Operator/2
  Switch3/1 -> Switch2/3
  Switch1/1 -> DEMd_enum_CtrCmd/1  "DEMd_enum_CtrCmd"
  Switch2/1 -> Switch1/3
  Relational Operator/1 -> Switch1/2
  DEMd_enum_DrvCtrCmd/1 -> Switch3/1
  BSCd_enum_BCUSt/1 -> Relational Operator2/1, Relational Operator1/1, Relational Operator/1

== system DEM_lib/Diagnostic_Event_Management/Level_handle/DRIVE ==
  DEMd_cflt_fault : Inport
  IPTd_flg_VehHVCnctCmd : Inport  Port=2
  BSCd_enum_BCUSt : Inport  Port=3
  FaultLevelConfirmed : Subsystem  Description=|
      | $Author:Yan LiJuan$
      | $Date:2015/03/26$  
      | $Revision:1.0$
  handle : Subsystem  Description=|
      | $Author:Yan LiJuan$
      | $Date:2015/03/26$  
      | $Revision:1.0$
  DEMd_enum_FaultLev : Outport
  DEMd_flg_TmOverWarn : Outport  Port=2
  DEMd_flg_HVdcnctReq : Outport  Port=3
  DEMd_enum_DrvCtrCmdRaw : Outport  Port=4
  wires:
  handle/3(DEMd_flg_TmOverWarn) -> DEMd_flg_TmOverWarn/1
  handle/2(DEMd_flg_HVdcnctReq) -> DEMd_flg_HVdcnctReq/1
  handle/1(DEMd_enum_CtrCmdRaw) -> DEMd_enum_DrvCtrCmdRaw/1
  BSCd_enum_BCUSt/1 -> handle/4(BSCd_enum_BCUSt)
  IPTd_flg_VehHVCnctCmd/1 -> handle/3(IPTd_flg_VehHVCnctCmd)
  FaultLevelConfirmed/1(DEMd_enum_FaultLev) -> handle/1(DEMd_enum_FaultLev), DEMd_enum_FaultLev/1
  DEMd_cflt_fault/1 -> handle/2(DEMd_cflt_fault), FaultLevelConfirmed/1(DEMd_cflt_fault)

== system DEM_lib/Diagnostic_Event_Management/fault_collect/BAL_Fault_Confirmed ==
  FaultBusAll_IN : Inport
  BALd_iflit_BalSwthAnml_warn : Inport  Port=2
  Bus Assignment : BusAssignment  Description=|  AssignedSignals=BAL_Fault_Bus.BALd_cflt_BalSwthAnml_warnRaw
      | $Author:Yan LiJuan$
      | $Date:2015/03/26$  
      | $Revision:1.0$
  Subsystem2 : Subsystem
  BALFaultBusAll_OUT : Outport
  wires:
  Subsystem2/1(cfault) -> Bus Assignment/2  "BALd_cflt_BalSwthAnml_warn"
  Bus Assignment/1 -> BALFaultBusAll_OUT/1
  BALd_iflit_BalSwthAnml_warn/1 -> Subsystem2/1(ifault)
  FaultBusAll_IN/1 -> Bus Assignment/1

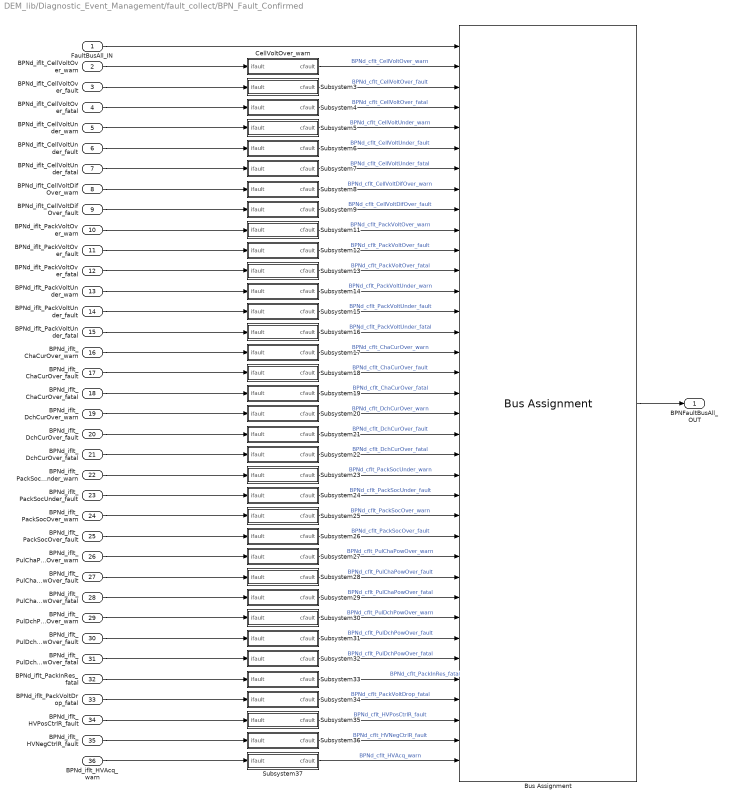
== system DEM_lib/Diagnostic_Event_Management/fault_collect/BPN_Fault_Confirmed ==
  FaultBusAll_IN : Inport
  BPNd_iflt_CellVoltOver_warn : Inport  Port=2
  BPNd_iflt_CellVoltOver_fault : Inport  Port=3
  BPNd_iflt_CellVoltOver_fatal : Inport  Port=4
  BPNd_iflt_CellVoltUnder_warn : Inport  Port=5
  BPNd_iflt_CellVoltUnder_fault : Inport  Port=6
  BPNd_iflt_CellVoltUnder_fatal : Inport  Port=7
  BPNd_iflt_CellVoltDifOver_warn : Inport  Port=8
  BPNd_iflt_CellVoltDifOver_fault : Inport  Port=9
  BPNd_iflt_PackVoltOver_warn : Inport  Port=10
  BPNd_iflt_PackVoltOver_fault : Inport  Port=11
  BPNd_iflt_PackVoltOver_fatal : Inport  Port=12
  BPNd_iflt_PackVoltUnder_warn : Inport  Port=13
  BPNd_iflt_PackVoltUnder_fault : Inport  Port=14
  BPNd_iflt_PackVoltUnder_fatal : Inport  Port=15
  BPNd_iflt_ChaCurOver_warn : Inport  Port=16
  BPNd_iflt_ChaCurOver_fault : Inport  Port=17
  BPNd_iflt_ChaCurOver_fatal : Inport  Port=18
  BPNd_iflt_DchCurOver_warn : Inport  Port=19
  BPNd_iflt_DchCurOver_fault : Inport  Port=20
  BPNd_iflt_DchCurOver_fatal : Inport  Port=21
  BPNd_iflt_PackSocUnder_warn : Inport  Port=22
  BPNd_iflt_PackSocUnder_fault : Inport  Port=23
  BPNd_iflt_PackSocOver_warn : Inport  Port=24
  BPNd_iflt_PackSocOver_fault : Inport  Port=25
  BPNd_iflt_PulChaPowOver_warn : Inport  Port=26
  BPNd_iflt_PulChaPowOver_fault : Inport  Port=27
  BPNd_iflt_PulChaPowOver_fatal : Inport  Port=28
  BPNd_iflt_PulDchPowOver_warn : Inport  Port=29
  BPNd_iflt_PulDchPowOver_fault : Inport  Port=30
  BPNd_iflt_PulDchPowOver_fatal : Inport  Port=31
  BPNd_iflt_PackInRes_fatal : Inport  Port=32
  BPNd_iflt_PackVoltDrop_fatal : Inport  Port=33
  BPNd_iflt_HVPosCtrlR_fault : Inport  Port=34
  BPNd_iflt_HVNegCtrlR_fault : Inport  Port=35
  BPNd_iflt_HVAcq_warn : Inport  Port=36
  Bus Assignment : BusAssignment  Description=|  AssignedSignals=BPN_Fault_Bus.BPNd_cflt_CellVoltOver_warnRaw,BPN_Fault_Bus.BPNd_cflt_CellVoltOver_faultRaw,BPN_Fault_Bus.BPNd_cflt_CellVoltOver_fatalRaw,BPN_Fault_Bus.BPNd_cflt_CellVoltUnder_warnRaw,BPN_Fault_Bus.BPNd_cflt_CellVoltUnder_faultRaw,BPN_Fault_Bus.BPNd_cflt_CellVoltUnder_fatalRaw,BPN_Fault_Bus.BPNd_cflt_CellVoltDifOver_warnRaw,BPN_Fault_Bus.BPNd_cflt_CellVoltDifOver_faultRaw,BPN_Fault_Bus.BPNd_cflt_PackVoltOver_warnRaw,BPN_Fault_Bus.BPNd_cflt_PackVoltOver_faultRaw,BPN_Fault_Bus.BPNd_cflt_PackVoltOver_fatalRaw,BPN_Fault_Bus.BPNd_cflt_PackVoltUnder_warnRaw,BPN_Fault_Bus.BPNd_cflt_PackVoltUnder_faultRaw,BPN_Fault_Bus.BPNd_cflt_PackVoltUnder_fatalRaw,BPN_Fault_Bus.BPNd_cflt_ChaCurOver_warnRaw,BPN_Fault_Bus.BPNd_cflt_ChaCurOver_faultRaw,BPN_Fault_Bus.BPNd_cflt_ChaCurOver_fatalRaw,BPN_Fault_Bus.BPNd_cflt_DchCurOver_warnRaw,BPN_Fault_Bus.BPNd_cflt_DchCurOver_faultRaw,BPN_Fault_Bus.BPNd_cflt_DchCurOver_fatalRaw,BPN_Fault_Bus.BPNd_cflt_PackSocUnder_warnRaw,BPN_Fault_Bus.BPNd_cflt_PackSocUnder_faultRaw,BPN_Fault_Bus.BPNd_cflt_PackSocOver_warnRaw,BPN_Fault_Bus.BPNd_cflt_PackSocOver_faultRaw,BPN_Fault_Bus.BPNd_cflt_PulChaPowOver_warnRaw,BPN_Fault_Bus.BPNd_cflt_PulChaPowOver_faultRaw,BPN_Fault_Bus.BPNd_cflt_PulChaPowOver_fatalRaw,BPN_Fault_Bus.BPNd_cflt_PulDchPowOver_warnRaw,BPN_Fault_Bus.BPNd_cflt_PulDchPowOver_faultRaw,BPN_Fault_Bus.BPNd_cflt_PulDchPowOver_fatalRaw,BPN_Fault_Bus.BPNd_cflt_PackInRes_fatalRaw,BPN_Fault_Bus.BPNd_cflt_PackVoltDrop_fatalRaw,BPN_Fault_Bus.BPNd_cflt_HVPosCtrlR_faultRaw,BPN_Fault_Bus.BPNd_cflt_HVNegCtrlR_faultRaw,BPN_Fault_Bus.BPNd_cflt_HVAcq_warnRaw
      | $Author:Yan LiJuan$
      | $Date:2015/03/26$  
      | $Revision:1.0$
  CellVoltOver_warn : Subsystem  Description=|
      | $Author:Yan LiJuan$
      | $Date:2015/03/26$  
      | $Revision:1.0$
  Subsystem11 : Subsystem
  Subsystem12 : Subsystem
  Subsystem13 : Subsystem
  Subsystem14 : Subsystem
  Subsystem15 : Subsystem
  Subsystem16 : Subsystem
  Subsystem17 : Subsystem
  Subsystem18 : Subsystem
  Subsystem19 : Subsystem
  Subsystem20 : Subsystem
  Subsystem21 : Subsystem
  Subsystem22 : Subsystem
  Subsystem23 : Subsystem
  Subsystem24 : Subsystem
  Subsystem25 : Subsystem
  Subsystem26 : Subsystem
  Subsystem27 : Subsystem
  Subsystem28 : Subsystem
  Subsystem29 : Subsystem
  Subsystem3 : Subsystem
  Subsystem30 : Subsystem
  Subsystem31 : Subsystem
  Subsystem32 : Subsystem
  Subsystem33 : Subsystem
  Subsystem34 : Subsystem
  Subsystem35 : Subsystem
  Subsystem36 : Subsystem
  Subsystem37 : Subsystem
  Subsystem4 : Subsystem
  Subsystem5 : Subsystem
  Subsystem6 : Subsystem
  Subsystem7 : Subsystem
  Subsystem8 : Subsystem
  Subsystem9 : Subsystem
  BPNFaultBusAll_OUT : Outport  OutDataType=fixdt(1, 16)  OutScaling=2^0
  wires:
  Subsystem34/1(cfault) -> Bus Assignment/33  "BPNd_cflt_PackVoltDrop_fatal"
  Subsystem37/1(cfault) -> Bus Assignment/36  "BPNd_cflt_HVAcq_warn"
  Subsystem36/1(cfault) -> Bus Assignment/35  "BPNd_cflt_HVNegCtrlR_fault"
  Subsystem35/1(cfault) -> Bus Assignment/34  "BPNd_cflt_HVPosCtrlR_fault"
  Subsystem33/1(cfault) -> Bus Assignment/32  "BPNd_cflt_PackInRes_fatal"
  Subsystem32/1(cfault) -> Bus Assignment/31  "BPNd_cflt_PulDchPowOver_fatal"
  Subsystem31/1(cfault) -> Bus Assignment/30  "BPNd_cflt_PulDchPowOver_fault"
  Subsystem30/1(cfault) -> Bus Assignment/29  "BPNd_cflt_PulDchPowOver_warn"
  Subsystem29/1(cfault) -> Bus Assignment/28  "BPNd_cflt_PulChaPowOver_fatal"
  Subsystem28/1(cfault) -> Bus Assignment/27  "BPNd_cflt_PulChaPowOver_fault"
  Subsystem27/1(cfault) -> Bus Assignment/26  "BPNd_cflt_PulChaPowOver_warn"
  Subsystem26/1(cfault) -> Bus Assignment/25  "BPNd_cflt_PackSocOver_fault"
  Subsystem25/1(cfault) -> Bus Assignment/24  "BPNd_cflt_PackSocOver_warn"
  Subsystem24/1(cfault) -> Bus Assignment/23  "BPNd_cflt_PackSocUnder_fault"
  Subsystem23/1(cfault) -> Bus Assignment/22  "BPNd_cflt_PackSocUnder_warn"
  Subsystem22/1(cfault) -> Bus Assignment/21  "BPNd_cflt_DchCurOver_fatal"
  Subsystem21/1(cfault) -> Bus Assignment/20  "BPNd_cflt_DchCurOver_fault"
  Subsystem20/1(cfault) -> Bus Assignment/19  "BPNd_cflt_DchCurOver_warn"
  Subsystem19/1(cfault) -> Bus Assignment/18  "BPNd_cflt_ChaCurOver_fatal"
  Subsystem18/1(cfault) -> Bus Assignment/17  "BPNd_cflt_ChaCurOver_fault"
  Subsystem17/1(cfault) -> Bus Assignment/16  "BPNd_cflt_ChaCurOver_warn"
  Subsystem16/1(cfault) -> Bus Assignment/15  "BPNd_cflt_PackVoltUnder_fatal"
  Subsystem15/1(cfault) -> Bus Assignment/14  "BPNd_cflt_PackVoltUnder_fault"
  Subsystem14/1(cfault) -> Bus Assignment/13  "BPNd_cflt_PackVoltUnder_warn"
  Subsystem13/1(cfault) -> Bus Assignment/12  "BPNd_cflt_PackVoltOver_fatal"
  Subsystem12/1(cfault) -> Bus Assignment/11  "BPNd_cflt_PackVoltOver_fault"
  Subsystem11/1(cfault) -> Bus Assignment/10  "BPNd_cflt_PackVoltOver_warn"
  Subsystem9/1(cfault) -> Bus Assignment/9  "BPNd_cflt_CellVoltDifOver_fault"
  Subsystem8/1(cfault) -> Bus Assignment/8  "BPNd_cflt_CellVoltDifOver_warn"
  Subsystem7/1(cfault) -> Bus Assignment/7  "BPNd_cflt_CellVoltUnder_fatal"
  Subsystem6/1(cfault) -> Bus Assignment/6  "BPNd_cflt_CellVoltUnder_fault"
  Subsystem5/1(cfault) -> Bus Assignment/5  "BPNd_cflt_CellVoltUnder_warn"
  Subsystem4/1(cfault) -> Bus Assignment/4  "BPNd_cflt_CellVoltOver_fatal"
  Subsystem3/1(cfault) -> Bus Assignment/3  "BPNd_cflt_CellVoltOver_fault"
  CellVoltOver_warn/1(cfault) -> Bus Assignment/2  "BPNd_cflt_CellVoltOver_warn"
  Bus Assignment/1 -> BPNFaultBusAll_OUT/1
  FaultBusAll_IN/1 -> Bus Assignment/1
  BPNd_iflt_PackVoltUnder_fault/1 -> Subsystem15/1(ifault)
  BPNd_iflt_HVAcq_warn/1 -> Subsystem37/1(ifault)
  BPNd_iflt_HVNegCtrlR_fault/1 -> Subsystem36/1(ifault)
  BPNd_iflt_HVPosCtrlR_fault/1 -> Subsystem35/1(ifault)
  BPNd_iflt_PackVoltDrop_fatal/1 -> Subsystem34/1(ifault)
  BPNd_iflt_PackInRes_fatal/1 -> Subsystem33/1(ifault)
  BPNd_iflt_PulDchPowOver_fatal/1 -> Subsystem32/1(ifault)
  BPNd_iflt_PulDchPowOver_fault/1 -> Subsystem31/1(ifault)
  BPNd_iflt_PulDchPowOver_warn/1 -> Subsystem30/1(ifault)
  BPNd_iflt_PulChaPowOver_fatal/1 -> Subsystem29/1(ifault)
  BPNd_iflt_PulChaPowOver_fault/1 -> Subsystem28/1(ifault)
  BPNd_iflt_PulChaPowOver_warn/1 -> Subsystem27/1(ifault)
  BPNd_iflt_PackSocOver_fault/1 -> Subsystem26/1(ifault)
  BPNd_iflt_PackSocOver_warn/1 -> Subsystem25/1(ifault)
  BPNd_iflt_PackSocUnder_fault/1 -> Subsystem24/1(ifault)
  BPNd_iflt_PackSocUnder_warn/1 -> Subsystem23/1(ifault)
  BPNd_iflt_DchCurOver_fatal/1 -> Subsystem22/1(ifault)
  BPNd_iflt_DchCurOver_fault/1 -> Subsystem21/1(ifault)
  BPNd_iflt_DchCurOver_warn/1 -> Subsystem20/1(ifault)
  BPNd_iflt_ChaCurOver_fatal/1 -> Subsystem19/1(ifault)
  BPNd_iflt_ChaCurOver_fault/1 -> Subsystem18/1(ifault)
  BPNd_iflt_ChaCurOver_warn/1 -> Subsystem17/1(ifault)
  BPNd_iflt_PackVoltUnder_fatal/1 -> Subsystem16/1(ifault)
  BPNd_iflt_PackVoltUnder_warn/1 -> Subsystem14/1(ifault)
  BPNd_iflt_PackVoltOver_fatal/1 -> Subsystem13/1(ifault)
  BPNd_iflt_PackVoltOver_fault/1 -> Subsystem12/1(ifault)
  BPNd_iflt_PackVoltOver_warn/1 -> Subsystem11/1(ifault)
  BPNd_iflt_CellVoltDifOver_fault/1 -> Subsystem9/1(ifault)
  BPNd_iflt_CellVoltDifOver_warn/1 -> Subsystem8/1(ifault)
  BPNd_iflt_CellVoltUnder_fatal/1 -> Subsystem7/1(ifault)
  BPNd_iflt_CellVoltUnder_fault/1 -> Subsystem6/1(ifault)
  BPNd_iflt_CellVoltUnder_warn/1 -> Subsystem5/1(ifault)
  BPNd_iflt_CellVoltOver_fatal/1 -> Subsystem4/1(ifault)
  BPNd_iflt_CellVoltOver_fault/1 -> Subsystem3/1(ifault)
  BPNd_iflt_CellVoltOver_warn/1 -> CellVoltOver_warn/1(ifault)

== system DEM_lib/Diagnostic_Event_Management/fault_collect/BSC_Fault_Confirmed ==
  FaultBusAll_IN : Inport
  BSCd_iflt_BCUFault : Inport  Port=2
  Bus Assignment : BusAssignment  Description=|  AssignedSignals=BSC_Fault_Bus.BSCd_cflt_BCUFaultRaw
      | $Author:Yan LiJuan$
      | $Date:2015/03/26$  
      | $Revision:1.0$
  Subsystem2 : Subsystem
  BSCFaultBusAll_OUT : Outport
  wires:
  Subsystem2/1(cfault) -> Bus Assignment/2  "BSCd_cflt_BCUFault"
  BSCd_iflt_BCUFault/1 -> Subsystem2/1(ifault)
  Bus Assignment/1 -> BSCFaultBusAll_OUT/1  "BSCFaultBusAll_OUT"
  FaultBusAll_IN/1 -> Bus Assignment/1

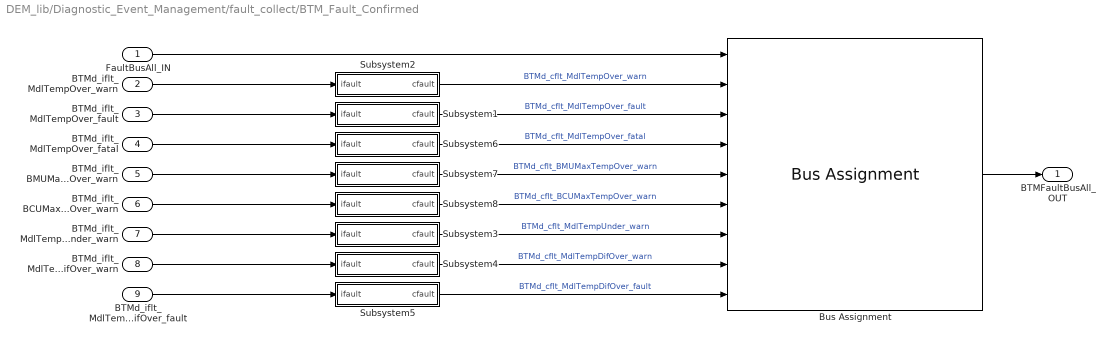
== system DEM_lib/Diagnostic_Event_Management/fault_collect/BTM_Fault_Confirmed ==
  FaultBusAll_IN : Inport
  BTMd_iflt_MdlTempOver_warn : Inport  Port=2
  BTMd_iflt_MdlTempOver_fault : Inport  Port=3
  BTMd_iflt_MdlTempOver_fatal : Inport  Port=4
  BTMd_iflt_BMUMaxTempOver_warn : Inport  Port=5
  BTMd_iflt_BCUMaxTempOver_warn : Inport  Port=6
  BTMd_iflt_MdlTempUnder_warn : Inport  Port=7
  BTMd_iflt_MdlTempDifOver_warn : Inport  Port=8
  BTMd_iflt_MdlTempDifOver_fault : Inport  Port=9
  Bus Assignment : BusAssignment  Description=|  AssignedSignals=BTM_Fault_Bus.BTMd_cflt_MdlTempOver_warnRaw,BTM_Fault_Bus.BTMd_cflt_MdlTempOver_faultRaw,BTM_Fault_Bus.BTMd_cflt_MdlTempOver_fatalRaw,BTM_Fault_Bus.BTMd_cflt_BMUMaxTempOver_warnRaw,BTM_Fault_Bus.BTMd_cflt_BCUMaxTempOver_warnRaw,BTM_Fault_Bus.BTMd_cflt_MdlTempUnder_warnRaw,BTM_Fault_Bus.BTMd_cflt_MdlTempDifOver_warnRaw,BTM_Fault_Bus.BTMd_cflt_MdlTempDifOver_faultRaw
      | $Author:Yan LiJuan$
      | $Date:2015/03/26$  
      | $Revision:1.0$
  Subsystem1 : Subsystem
  Subsystem2 : Subsystem
  Subsystem3 : Subsystem
  Subsystem4 : Subsystem
  Subsystem5 : Subsystem
  Subsystem6 : Subsystem
  Subsystem7 : Subsystem
  Subsystem8 : Subsystem
  BTMFaultBusAll_OUT : Outport
  wires:
  Subsystem8/1(cfault) -> Bus Assignment/6  "BTMd_cflt_BCUMaxTempOver_warn"
  Subsystem7/1(cfault) -> Bus Assignment/5  "BTMd_cflt_BMUMaxTempOver_warn"
  Subsystem6/1(cfault) -> Bus Assignment/4  "BTMd_cflt_MdlTempOver_fatal"
  Subsystem5/1(cfault) -> Bus Assignment/9  "BTMd_cflt_MdlTempDifOver_fault"
  Subsystem4/1(cfault) -> Bus Assignment/8  "BTMd_cflt_MdlTempDifOver_warn"
  Subsystem3/1(cfault) -> Bus Assignment/7  "BTMd_cflt_MdlTempUnder_warn"
  BTMd_iflt_BCUMaxTempOver_warn/1 -> Subsystem8/1(ifault)
  BTMd_iflt_BMUMaxTempOver_warn/1 -> Subsystem7/1(ifault)
  BTMd_iflt_MdlTempOver_fatal/1 -> Subsystem6/1(ifault)
  Subsystem1/1(cfault) -> Bus Assignment/3  "BTMd_cflt_MdlTempOver_fault"
  Subsystem2/1(cfault) -> Bus Assignment/2  "BTMd_cflt_MdlTempOver_warn"
  BTMd_iflt_MdlTempDifOver_fault/1 -> Subsystem5/1(ifault)
  BTMd_iflt_MdlTempDifOver_warn/1 -> Subsystem4/1(ifault)
  BTMd_iflt_MdlTempUnder_warn/1 -> Subsystem3/1(ifault)
  BTMd_iflt_MdlTempOver_fault/1 -> Subsystem1/1(ifault)
  BTMd_iflt_MdlTempOver_warn/1 -> Subsystem2/1(ifault)
  Bus Assignment/1 -> BTMFaultBusAll_OUT/1
  FaultBusAll_IN/1 -> Bus Assignment/1

== system DEM_lib/Diagnostic_Event_Management/fault_collect/COR_Fault_Confirmed ==
  FaultBusAll_IN : Inport
  CORd_iflt_CellCDcse_fault : Inport  Port=2
  CORd_iflt_CellRDcse_fault : Inport  Port=3
  CORd_iflt_CellRIcse_fault : Inport  Port=4
  Bus Assignment : BusAssignment  Description=|  AssignedSignals=COR_Fault_Bus.CORd_cflt_CellCDcse_faultRaw,COR_Fault_Bus.CORd_cflt_CellRDcse_faultRaw,COR_Fault_Bus.CORd_cflt_CellRIcse_faultRaw
      | $Author:Yan LiJuan$
      | $Date:2015/03/26$  
      | $Revision:1.0$
  Subsystem1 : Subsystem
  Subsystem5 : Subsystem
  Subsystem8 : Subsystem
  CORFaultBusAll_OUT : Outport
  wires:
  Subsystem8/1(cfault) -> Bus Assignment/4  "CORd_cflt_CellRIcse_fault"
  Subsystem5/1(cfault) -> Bus Assignment/3  "CORd_cflt_CellRDcse_fault"
  Subsystem1/1(cfault) -> Bus Assignment/2  "CORd_cflt_CellCDcse_fault"
  Bus Assignment/1 -> CORFaultBusAll_OUT/1
  CORd_iflt_CellRIcse_fault/1 -> Subsystem8/1(ifault)
  CORd_iflt_CellRDcse_fault/1 -> Subsystem5/1(ifault)
  CORd_iflt_CellCDcse_fault/1 -> Subsystem1/1(ifault)
  FaultBusAll_IN/1 -> Bus Assignment/1
